simulink model "simulation"  (R2023a)
settings: Solver=FixedStepAuto  StartTime=0.0  StopTime=3  FixedStep=Ts  RelTol=1e-3
values from neighbouring files (symbols this model uses):
  Dz = tf(num, den, Ts)    [controllers.m]    (also in dpidfun.m)
  G = tf(K, [tau 1], 'InputDelay', theta)    [FOD.m]    (also in controllers.m = Gs)
  Gd = Gsd    [controllers.m]
  inflim = 15    [controllers.m]
  maxlim = 80    [controllers.m]
libraries: simulink x1
settings Model: Creator=DANIEL  LastModifiedBy=DANIEL
settings SolverCC: ConcurrentTasks=on  PositivePriorityOrder=on
settings OptimizationCC: BlockReduction=off  OptimizeBlockIOStorage=off
settings DebuggingCC: TasksWithSamePriorityMsg=none
settings HardwareCC: ProdBitPerLong=64  ProdLongLongMode=on  ProdHWDeviceType=Intel->x86-64 (Linux 64)
settings RTWCC: Description=Simulink Real-Time  SystemTargetFile=slrealtime.tlc  TemplateMakefile=slrealtime_default_tmf  Toolchain=Simulink Real-Time Toolchain  BuildConfiguration=Faster Runs  CodeExecutionProfiling=on  TargetLang=C++

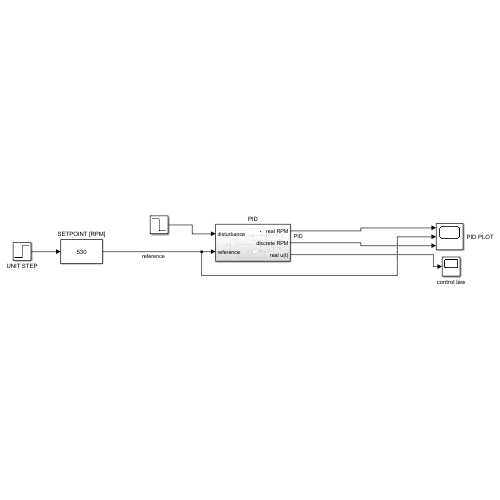
[thumbnail: Simulink's stored preview of the top-level diagram]
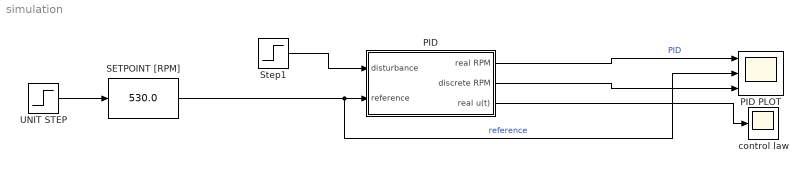
== system simulation ==
  PID : Subsystem
  PID PLOT : Scope  NumInputPorts=3
  SETPOINT [RPM] : simulink/Math Operations/Slider Gain  gain=530.0  low=0  high=1000
  Step1 : Step  Time=1.5  After=-7  SampleTime=0
  UNIT STEP : Step  Time=0  SampleTime=0
  control law : Scope
  wires:
  SETPOINT [RPM]/1 -> PID PLOT/2, PID/2(reference)  "reference"
  UNIT STEP/1 -> SETPOINT [RPM]/1
  PID/1(real RPM) -> PID PLOT/1  "PID"
  PID/2(discrete RPM) -> PID PLOT/3
  PID/3(real u(t)) -> control law/1
  Step1/1 -> PID/1(disturbance)

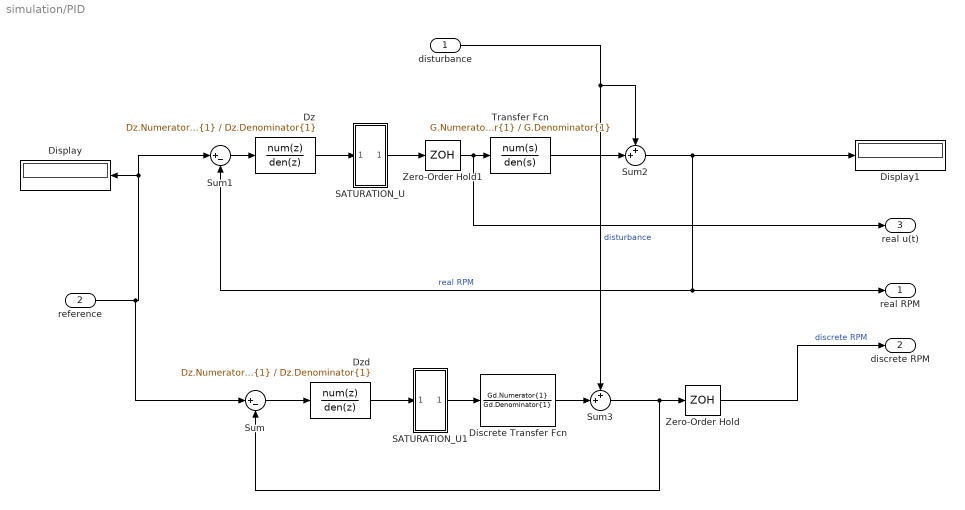
== system simulation/PID ==
  disturbance : Inport
  reference : Inport  Port=2
  Discrete Transfer Fcn : DiscreteTransferFcn  Numerator=Gd.Numerator{1}  Denominator=Gd.Denominator{1}
  Display : Display
  Display1 : Display
  Dz : DiscreteTransferFcn  Numerator=Dz.Numerator{1}  Denominator=Dz.Denominator{1}
  Dzd : DiscreteTransferFcn  Numerator=Dz.Numerator{1}  Denominator=Dz.Denominator{1}
  SATURATION_U : Subsystem
  SATURATION_U1 : Subsystem
  Sum : Sum  Inputs=|+-
  Sum1 : Sum  Inputs=|+-
  Sum2 : Sum  Inputs=++|
  Sum3 : Sum  Inputs=++|
  Transfer Fcn : TransferFcn  Numerator=G.Numerator{1}  Denominator=G.Denominator{1}
  Zero-Order Hold : ZeroOrderHold  SampleTime=-1
  Zero-Order Hold1 : ZeroOrderHold  SampleTime=-1
  real RPM : Outport
  discrete RPM : Outport  Port=2
  real u(t) : Outport  Port=3
  wires:
  Sum2/1 -> Display1/1, Sum1/2, real RPM/1  "real RPM"
  Dzd/1 -> SATURATION_U1/1(In1)
  Sum/1 -> Dzd/1
  disturbance/1 -> Sum2/1, Sum3/1  "disturbance"
  Sum1/1 -> Dz/1
  Discrete Transfer Fcn/1 -> Sum3/2
  reference/1 -> Sum/1, Sum1/1, Display/1
  Dz/1 -> SATURATION_U/1(In1)
  Transfer Fcn/1 -> Sum2/2
  Sum3/1 -> Sum/2, Zero-Order Hold/1
  Zero-Order Hold1/1 -> real u(t)/1, Transfer Fcn/1
  Zero-Order Hold/1 -> discrete RPM/1  "discrete RPM"
  SATURATION_U1/1(Out1) -> Discrete Transfer Fcn/1
  SATURATION_U/1(Out1) -> Zero-Order Hold1/1

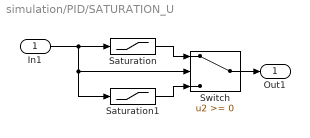
== system simulation/PID/SATURATION_U ==
  In1 : Inport
  Saturation : Saturate  UpperLimit=maxlim  LowerLimit=inflim
  Saturation1 : Saturate  UpperLimit=-inflim  LowerLimit=-maxlim
  Switch : Switch  SaturateOnIntegerOverflow=off  InputSameDT=off
  Out1 : Outport
  wires:
  Switch/1 -> Out1/1
  Saturation1/1 -> Switch/3
  Saturation/1 -> Switch/1
  In1/1 -> Switch/2, Saturation1/1, Saturation/1

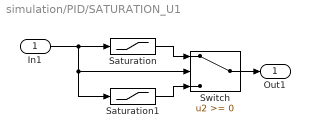
== system simulation/PID/SATURATION_U1 ==
  In1 : Inport
  Saturation : Saturate  UpperLimit=maxlim  LowerLimit=inflim
  Saturation1 : Saturate  UpperLimit=-inflim  LowerLimit=-maxlim
  Switch : Switch  SaturateOnIntegerOverflow=off  InputSameDT=off
  Out1 : Outport
  wires:
  In1/1 -> Saturation/1, Saturation1/1, Switch/2
  Saturation/1 -> Switch/1
  Saturation1/1 -> Switch/3
  Switch/1 -> Out1/1
